simulink model "W8_Stateflow_PC_2020b"  (R2021b)
settings: Solver=FixedStepAuto  StartTime=0.0  StopTime=inf  RelTol=1e-3  EnableMultiTasking=on
libraries: arduinolib x3, arduinosensorlib x1
settings Model: ExtModeTrigDuration=2  Creator=yitwang6  LastModifiedBy=yitin
settings SolverCC: AlgebraicLoopSolver=TrustRegion
settings OptimizationCC: EnhancedBackFolding=on  PassReuseOutputArgsThreshold=0  MaxStackSize=64  OptimizeBlockOrder=speed  DifferentSizesBufferReuse=on  OptimizationCustomize=off
settings DebuggingCC: ParameterTunabilityLossMsg=error  SFMachineParentedDataDiag=warning
settings HardwareCC: ProdBitPerInt=16  ProdBitPerPointer=16  ProdBitPerSizeT=16  ProdBitPerPtrDiffT=16  ProdLargestAtomicFloat=None  ProdWordSize=8  ProdHWDeviceType=Atmel->AVR  UseEmbeddedCoderFeatures=off
settings SFSimCC: MATLABDynamicMemAlloc=off
settings RTWCC: Description=Embedded Coder  SystemTargetFile=ert.tlc  HardwareBoard=Arduino Uno  TemplateMakefile=ert_default_tmf  Toolchain=Arduino AVR  BuildConfiguration=Faster Runs
settings CodeAppCC: ForceParamTrailComments=on  OperatorAnnotations=on
settings ERTTargetCC: ERTCustomFileBanners=off  SupportContinuousTime=on  SupportNonInlinedSFcns=on  RemoveResetFunc=off  SupportVariableSizeSignals=on  ModelStepFunctionPrototypeControlCompliant=off  ExtModeStaticAllocSize=250

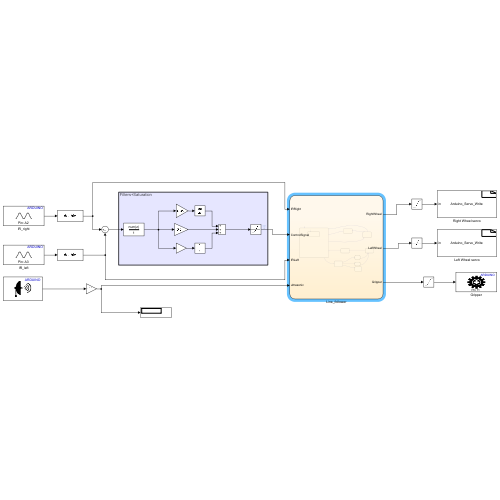
[thumbnail: Simulink's stored preview of the top-level diagram]
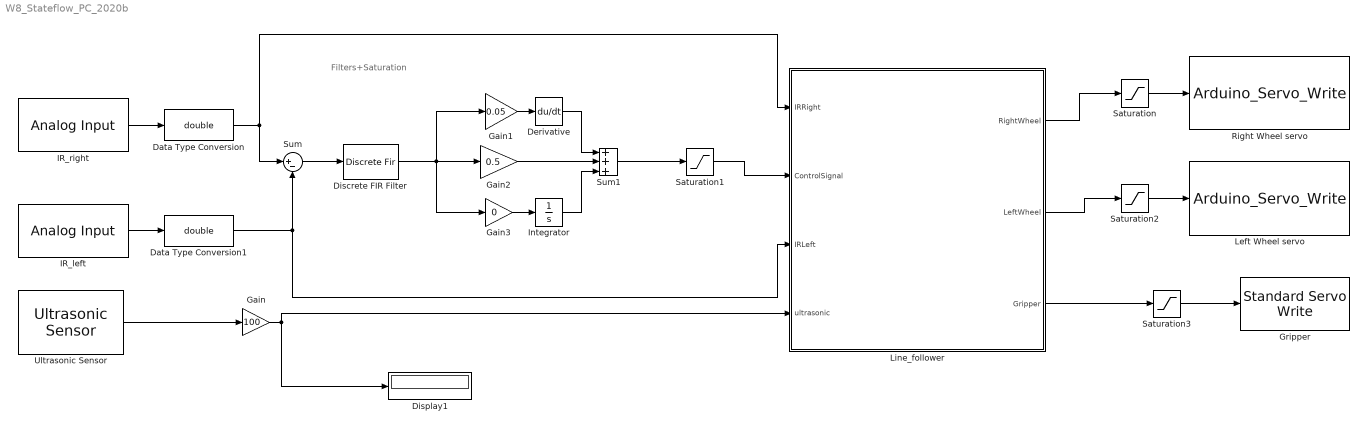
== system W8_Stateflow_PC_2020b ==
  note: Filters+Saturation
  Data Type Conversion : DataTypeConversion  OutDataTypeStr=double
  Data Type Conversion1 : DataTypeConversion  OutDataTypeStr=double
  Derivative : Derivative
  Discrete FIR Filter : DiscreteFir  Coefficients=[ones(1,25)/25]
  Display1 : Display
  Gain : Gain  Gain=100
  Gain1 : Gain  Gain=0.05
  Gain2 : Gain  Gain=0.5
  Gain3 : Gain  Gain=0
  Gripper : arduinolib/Standard Servo Write  pinNumber=11  ServoIndex=0  blockPlatform=ARDUINO
  IR_left : arduinolib/Analog Input  pinNumber=3  ReadResultsOnly=off  ConversionTriggerSource=Software  ExternalTriggerType=uint32( 0 )  OutputDataType=uint16  EnableConversionCompleteNotify=off  EnableOuputStatus=off  SampleTime=0.001  blockPlatform=arduino
  IR_right : arduinolib/Analog Input  pinNumber=2  ReadResultsOnly=off  ConversionTriggerSource=Software  ExternalTriggerType=uint32( 0 )  OutputDataType=uint16  EnableConversionCompleteNotify=off  EnableOuputStatus=off  SampleTime=0.001  blockPlatform=arduino
  Integrator : Integrator
  Left Wheel servo : S-Function  InitFcn=try, set_param(gcb,'FunctionName','Arduino_Servo_Write'), end  FunctionName=Arduino_Servo_Write  Parameters=int8(Pin)  SFunctionModules=Arduino_Servo_Write_wrapper  SFunctionDeploymentMode=off  EnableBusSupport=off  mask(Servo Write){Pin=13}
      mask prompts: Pin "Pin Number"
      mask help:
      | This block can be used to write to Continuous or Standard Servo.
      | The block will generate a HIGH signal of pulsewidth (microseconds) specified by the input followed by a 20ms LOW signal.
      |
      | Input:
      | - pulsewidth of 1500 for continuous servo with no rotation
      | - pulsewidth 1500 for standard servo center position
      mask init:
      | val = [[.9  0.75 0.75 1 1 .9 .9 1]',[1 1 0.75 0.75 .9 .9 1 .9]'];try , sys = get_param(gcb,'SfunBuilderFcnName');if isempty(sys), sys = get_param(gcb,'FunctionName'); end,catch, sys = get_param(gcb,'FunctionName'); end
      settings: CopyFcn=set_param(gcbh,'LinkStatus','none')  PreSaveFcn=try, set_param(gcb,'FunctionName','Arduino_Servo_Write'), end  OpenFcn=sfunctionwizard(gcbh)
      mask Display: plot(val(:,1),val(:,2)),disp(sys), port_label('input',1,'in')
  Line_follower : Stateflow chart  TreatAsAtomicUnit=on
  Right Wheel servo : S-Function  InitFcn=try, set_param(gcb,'FunctionName','Arduino_Servo_Write'), end  FunctionName=Arduino_Servo_Write  Parameters=int8(Pin)  SFunctionModules=Arduino_Servo_Write_wrapper  SFunctionDeploymentMode=off  EnableBusSupport=off  mask(Servo Write){Pin=12}
      mask prompts: Pin "Pin Number"
      mask help:
      | This block can be used to write to Continuous or Standard Servo.
      | The block will generate a HIGH signal of pulsewidth (microseconds) specified by the input followed by a 20ms LOW signal.
      |
      | Input:
      | - pulsewidth of 1500 for continuous servo with no rotation
      | - pulsewidth 1500 for standard servo center position
      mask init: same as W8_Stateflow_PC_2020b/Left Wheel servo
      settings: CopyFcn=set_param(gcbh,'LinkStatus','none')  PreSaveFcn=try, set_param(gcb,'FunctionName','Arduino_Servo_Write'), end  OpenFcn=sfunctionwizard(gcbh)
      mask Display: plot(val(:,1),val(:,2)),disp(sys), port_label('input',1,'in')
  Saturation : Saturate  UpperLimit=1600  LowerLimit=1400
  Saturation1 : Saturate  UpperLimit=100  LowerLimit=-100
  Saturation2 : Saturate  UpperLimit=1600  LowerLimit=1400
  Saturation3 : Saturate  UpperLimit=180  LowerLimit=80
  Sum : Sum  Inputs=|+-
  Sum1 : Sum  Inputs=|+|+|+|
  Ultrasonic Sensor : arduinosensorlib/Ultrasonic Sensor  NumSignalPins=1  TrigPin=4  EchoPin=5  SignalPin=9  SampleTime_=0.001  blockPlatform=ARDUINO
      settings: SourceProductBaseCode=ARDUINO
  wires:
  Data Type Conversion1/1 -> Sum/2, Line_follower/3(IRLeft)
  Line_follower/1(RightWheel) -> Saturation/1
  Gain/1 -> Line_follower/4(ultrasonic), Display1/1
  Ultrasonic Sensor/1 -> Gain/1
  IR_left/1 -> Data Type Conversion1/1
  Line_follower/2(LeftWheel) -> Saturation2/1
  Sum/1 -> Discrete FIR Filter/1
  IR_right/1 -> Data Type Conversion/1
  Data Type Conversion/1 -> Sum/1, Line_follower/1(IRRight)
  Line_follower/3(Gripper) -> Saturation3/1
  Discrete FIR Filter/1 -> Gain3/1, Gain2/1, Gain1/1
  Saturation/1 -> Right Wheel servo/1
  Saturation2/1 -> Left Wheel servo/1
  Saturation3/1 -> Gripper/1
  Saturation1/1 -> Line_follower/2(ControlSignal)
  Gain2/1 -> Sum1/2
  Sum1/1 -> Saturation1/1
  Gain1/1 -> Derivative/1
  Derivative/1 -> Sum1/1
  Gain3/1 -> Integrator/1
  Integrator/1 -> Sum1/3

== stateflow chart W8_Stateflow_PC_2020b/Line_follower ==
  state Driving
    state Drive_prop
      RightWheel = 1400-ControlSignal;
      LeftWheel = 1600-ControlSignal;
    (default) -> Drive_prop
  state Turn_Back_ultrasonic
    RightWheel = 1600;
    LeftWheel = 1600;
  state Stop_ultrasonic
    RightWheel = 1500;
    LeftWheel = 1500;
    Gripper = 95;
  state Turn_Back
    RightWheel = 1600;
    LeftWheel = 1600;
  state Back_Up
    RightWheel = 1600;
    LeftWheel = 1400;
  state Count1
    Count=1;
  state Stop
    RightWheel = 1500;
    LeftWheel = 1500;
    Gripper = 175;
  state Count2
    Count=2;
  state Count3
    RightWheel = 1500;
    LeftWheel = 1500;
  Stop_ultrasonic -> Driving [order 1] : [Count==2]
  (default) -> Driving : {Gripper = 180, Count=0}
  Stop_ultrasonic -> Turn_Back_ultrasonic [order 2] : after(0.08,sec)[Count<2]
  Turn_Back_ultrasonic -> Driving : [IRLeft > 800 && IRRight<700 && 40>=ControlSignal>=-40]
  Driving -> Stop_ultrasonic [order 2] : [ultrasonic<6 && Gripper ~= 95]
  Back_Up -> Turn_Back : after(0.01,sec)
  Turn_Back -> Driving : [IRLeft >800 && IRRight<700 && 40>=ControlSignal>=-40]
  Count1 -> Back_Up : after(0.02,sec)
  Count2 -> Back_Up : after(0.02,sec)
  Stop -> Count1 [order 1] : [Count==0]
  Driving -> Stop [order 1] : [IRLeft < 650 && IRRight<650 && 20>=ControlSignal>=-20]
  Stop -> Count2 [order 2] : [Count==1]
  Stop -> Count3 [order 3] : [Count==2]
  data: IRRight input; RightWheel output; LeftWheel output; ControlSignal input; IRLeft input; ultrasonic input; Gripper output; Count local
